simulink model "vis_test_model"  (R2026a)
settings: Solver=FixedStepDiscrete  StopTime=15  FixedStep=0.05
settings Model: Creator=anees  LastModifiedBy=anees

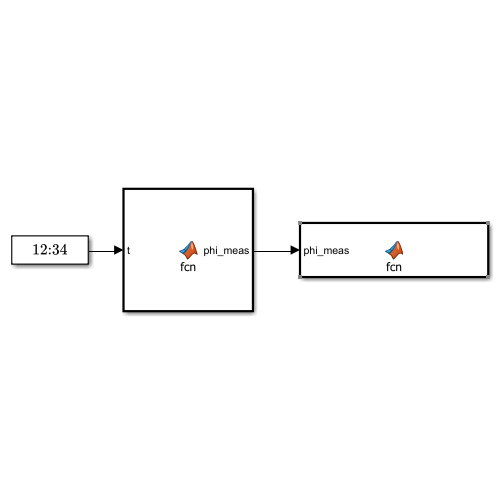
[thumbnail: Simulink's stored preview of the top-level diagram]
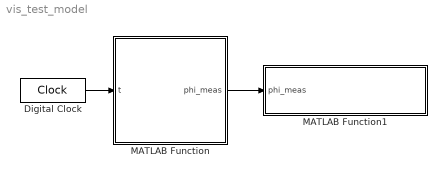
== system vis_test_model ==
  Digital Clock : DigitalClock  SampleTime=0.05
  MATLAB Function : MATLAB Function  TreatAsAtomicUnit=on
  MATLAB Function1 : MATLAB Function  TreatAsAtomicUnit=on
  wires:
  MATLAB Function/1(phi_meas) -> MATLAB Function1/1(phi_meas)
  Digital Clock/1 -> MATLAB Function/1(t)

== matlab function vis_test_model/MATLAB Function ==
  data: t input; phi_meas output
function phi_meas = fcn(t)
% Generate one ordered measurement at each simulation step.

phi_meas = zeros(4,1);

phi_meas(1) = 0;                              % base
phi_meas(2) = mod(0.4*t, 2*pi);              % shoulder
phi_meas(3) = pi/2 + (pi/3)*sin(0.8*t);      % elbow
phi_meas(4) = 0;                              % wrist
end

== matlab function vis_test_model/MATLAB Function1 ==
  data: phi_meas input
function fcn(phi_meas)
% MATLAB graphics are simulation-only.
coder.extrinsic('vis');

vis(phi_meas);
end
